simulink model "zcanreceivepot"  (R2018a)
settings: Solver=FixedStepDiscrete  StartTime=0.0  StopTime=10.0  FixedStep=0.1  RelTol=1e-3
InitFcn:
  | mbd_pnt_consistency_checks(bdroot(gcs));
undefined symbols (not defined in the file): A14, A15, A3, B0, B1, C14, C16, D3
libraries: mbd_pnt_ec_toolbox x3
settings Model: Creator=oolonthegreat  LastModifiedBy=oolonthegreat
settings DataIOCC: ExternalInput=off  InitialState=off  SaveOutput=off  SignalLogging=off  SaveTime=off
settings OptimizationCC: DefaultParameterBehavior=Inlined  EnhancedBackFolding=on  PassReuseOutputArgsAs=Individual arguments  OptimizeBlockOrder=speed  DifferentSizesBufferReuse=on  OptimizationCustomize=off
settings DebuggingCC: InheritedTsInSrcMsg=none  SingleTaskRateTransMsg=error  ParameterTunabilityLossMsg=error  UnconnectedInputMsg=error  UnconnectedOutputMsg=error  UnconnectedLineMsg=error  UnknownTsInhSupMsg=error
settings HardwareCC: ProdBitPerPointer=32  ProdBitPerSizeT=32  ProdBitPerPtrDiffT=32  ProdLargestAtomicInteger=Long  ProdLargestAtomicFloat=Double  ProdEndianess=BigEndian  ProdWordSize=32  ProdHWDeviceType=Motorola PowerPC
settings SFSimCC: MATLABDynamicMemAlloc=off
settings RTWCC: SystemTargetFile=mbd_pnt.tlc  MakeCommand=mbd_pnt_make_rtw COPY_MDLREF_INCLUDES=0  TemplateMakefile=mbd_pnt.tmf  PostCodeGenCommand=mbd_pnt_analyzegencode(buildInfo)  Description=Model Based Design Toolbox MPC574xP Code Generation Target  GenerateReport=on  IncludeHyperlinkInReport=on  LaunchReport=on  GenerateTraceInfo=on  GenerateTraceReport=on  GenerateTraceReportSl=on  GenerateTraceReportSf=on  GenerateTraceReportEml=on
settings CodeAppCC: ForceParamTrailComments=on  IgnoreCustomStorageClasses=off  OperatorAnnotations=on  SimulinkDataObjDesc=on  SFDataObjDesc=on  InsertBlockDesc=on
settings STFCustomTargetCC: TargetLangStandard=C99 (ISO)  MultiwordLength=256  CombineOutputUpdateFcns=on  SuppressErrorStatus=on  ERTCustomFileBanners=on  SupportContinuousTime=off  SupportNonInlinedSFcns=off  RemoveResetFunc=on  MATLABClassNameForMDSCustomization=Simulink.SoftwareTarget.ERTCustomization  GRTInterface=off  SystemTargetFile=mbd_pnt.tlc
settings ERTTargetCC: TargetLangStandard=C99 (ISO)  ParMdlRefBuildCompliant=off  CompOptLevelCompliant=off  ConcurrentExecutionCompliant=off  SuppressErrorStatus=on  ModelStepFunctionPrototypeControlCompliant=off  CPPClassGenCompliant=off  UseToolchainInfoCompliant=off  InlinedParameterPlacement=NonHierarchical  ERTCustomFileTemplate=example_file_process.tlc

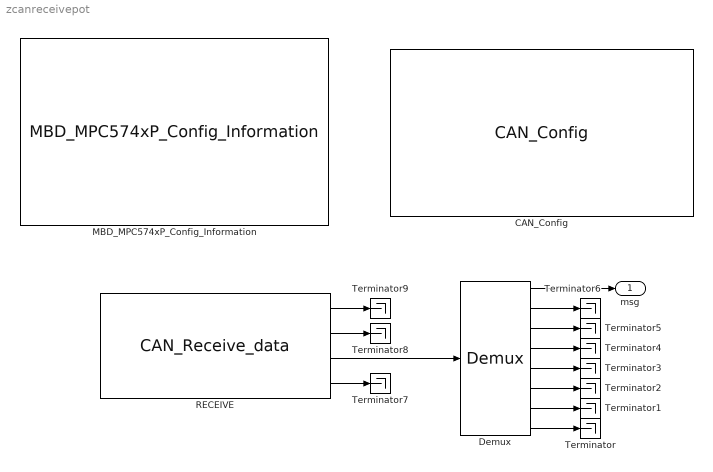
== system zcanreceivepot ==
  CAN_Config : mbd_pnt_ec_toolbox/MPC574xP/Communication Blocks/CAN_Config  Priority=1  can_unit=0  can_idam=A - One full ID (standard or extended) per filter element.  can_srx_dis=1 - Self reception disabled  can_presdiv=3  can_rjw=1  can_pseg1=1  can_pseg2=1  can_clk_src=1 - The CAN engine clock source is the bus clock  can_lpb=0 - Loop Back disabled  can_smp=1 - Three samples are used to determine the value of the received bit  can_boff_rec=0 - Automatic recovering from Bus Off state enabled  can_tsyn=0 - Timer Sync feature disabled  can_lbuf=0 - Buffer with highest priority is transmitted first  can_lom=0 - Listen Only Mode is deactivated  can_propseg=3  psr_RxD=17  psr_TxD=16  can0_RxD="17 : B1   : [110] : [135] : [C14]"  can0_TxD=16 : B0 : [109] : [134] : [C16]  can1_RxD=15 : A15 : [144] : [176] : [D3]  can1_TxD=14 : A14 : [143] : [175] : [A3]  can2_RxD=None  can2_TxD=None
      settings: SourceProductName=Model Based Design Toolbox for MPC574xP
  Demux : Demux  Outputs=8
  MBD_MPC574xP_Config_Information : mbd_pnt_ec_toolbox/MPC574xP/MBD_MPC574xP_Config_Information  disp_str=|  config_params=[]
      | System Clock : 200 MHz
      | Target : MPC5744P
      | Package : 144LQFP
      | XTAL Freq : 40 MHz
      | Compiler : S32 Design Studio
      | Target Type : FLASH
      | Global Interrupt Priority : 8
      | System Tick Interrupt Priority : 12
      | Freemaster : Serial1 (115200 Kbits)
      | Download Code after build : (COM5,115200)
      settings: SourceProductName=Model Based Design Toolbox for MPC574xP
  RECEIVE : mbd_pnt_ec_toolbox/MPC574xP/Communication Blocks/CAN_Receive_data  can_unit=0  can_buffer=0  can_id=1010
      settings: SourceProductName=Model Based Design Toolbox for MPC574xP
  Terminator{,1..9} (10 alike) : Terminator
  msg : Outport
  wires:
  RECEIVE/3 -> Demux/1
  Demux/2 -> Terminator6/1
  Demux/1 -> msg/1
  Demux/3 -> Terminator5/1
  Demux/4 -> Terminator4/1
  Demux/5 -> Terminator3/1
  Demux/6 -> Terminator2/1
  Demux/7 -> Terminator1/1
  Demux/8 -> Terminator/1
  RECEIVE/1 -> Terminator9/1
  RECEIVE/2 -> Terminator8/1
  RECEIVE/4 -> Terminator7/1
